simulink model "message_ros_deserialize_receive"  (R2020b)
settings: Solver=FixedStepAuto  StartTime=0.0  StopTime=inf  FixedStep=0.05  RelTol=1e-3
libraries: simulink x2, robotlib x1, ROSMessageSerializer x1, dspnetwork x1
settings Model: EnablePacing=on  Creator=jarisafi  LastModifiedBy=promero
settings SolverCC: InsertRTBMode=Never (minimum delay)
settings DataIOCC: SaveFormat=StructureWithTime  ReturnWorkspaceOutputs=off
settings OptimizationCC: BlockReduction=off  OptimizeBlockIOStorage=off  BufferReuse=off  GlobalBufferReuse=off  ExpressionFolding=off  LocalBlockOutputs=off
settings DebuggingCC: ArithmeticOperatorsInVariantConditions=warning
settings SFSimCC: SimUseLocalCustomCode=off  CustomCodeUndefinedFunction=UseInterfaceOnly
settings RTWCC: PackageName=packNgo_out.zip  RTWUseLocalCustomCode=off
settings CodeAppCC: StateflowObjectComments=on
settings GRTTargetCC: TargetLangStandard=C89/C90 (ANSI)

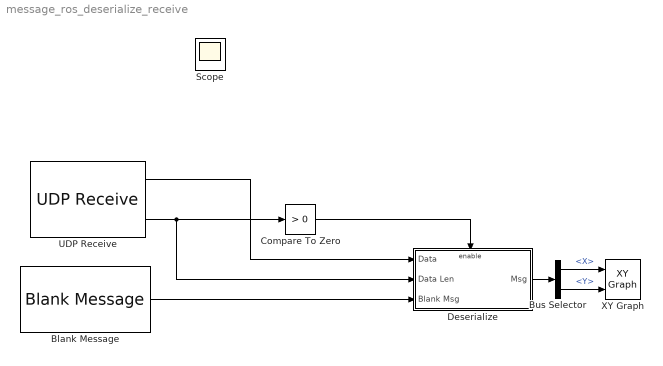
== system message_ros_deserialize_receive ==
  Blank Message : robotlib/Blank Message  messageClass=Message  entityType=nav_msgs/Odometry  messageType=nav_msgs/Odometry  SampleTime=inf  legacyBusStruct=off
  Bus Selector : BusSelector  OutputSignals=Pose.Pose.Position.X,Pose.Pose.Position.Y
  Compare To Zero : simulink/Logic and Bit Operations/Compare To Zero  relop=>  OutDataTypeStr=boolean
  Deserialize : Subsystem  TreatAsAtomicUnit=on
  UDP Receive : dspnetwork/UDP Receive  localURL='0.0.0.0'  localPort=25000  remoteURL='0.0.0.0'  remotePort=-1  recvBufferSize=8192  dims=8192  signalDatatype=uint8  isComplex=off  isVarSize=off  showBlockingTime=off  blockingTime=0  sampletime=0.1  blockPlatform=[]
  XY Graph : simulink/Sinks/XY Graph  xmin=-10  xmax=10  ymin=-10  ymax=10  st=-1
  Scope : Scope
  wires:
  Blank Message/1 -> Deserialize/3(Blank Msg)
  UDP Receive/2 -> Compare To Zero/1, Deserialize/2(Data Len)
  UDP Receive/1 -> Deserialize/1(Data)
  Compare To Zero/1 -> Deserialize/Enable
  Deserialize/1(Msg) -> Bus Selector/1
  Bus Selector/1 -> XY Graph/1  "<X>"
  Bus Selector/2 -> XY Graph/2  "<Y>"

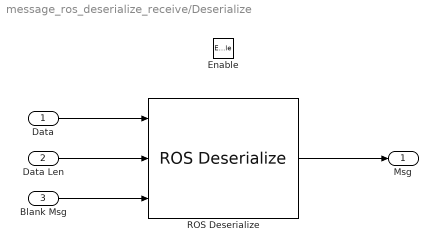
== system message_ros_deserialize_receive/Deserialize ==
  Data : Inport
  Data Len : Inport  Port=2
  Blank Msg : Inport  Port=3
  Enable : EnablePort  PropagateVarSize=During execution
  ROS Deserialize : ROSMessageSerializer/ROS Deserialize  MessageType=nav_msgs/Odometry  SimulateUsing=Code generation
      settings: SourceProductName=ROS/ROS2 Message (De)Serializer
  Msg : Outport
  wires:
  Data/1 -> ROS Deserialize/1
  ROS Deserialize/1 -> Msg/1
  Data Len/1 -> ROS Deserialize/2
  Blank Msg/1 -> ROS Deserialize/3
